simulink model "mainV02_36"  (R2016b)
settings: Solver=FixedStepAuto  StartTime=0.0  StopTime=inf  FixedStep=Ts  MaxStep=0.2  RelTol=1e-2
undefined symbols (not defined in the file): checks, deltae_degrees, deltafl_degrees, deltafr_degrees, deltar_degrees, deltat_1, deltat_2, deltat_3, deltat_4, deltat_5, Earth, F, ft, groundReaction, initialValues, LD, Light, m, MIL, Newton, Raphson, s, sigbuilder_block, Ts, WGS84
libraries: aerolibutil x19, simulink x16, aerolibtransform2 x7, aerolibasang x4, aerolib6dofsys x4, aerolib6dof2 x4, aerolibwind2 x3, aerolibbdyn x3, aerolibconvert2 x3, aerolibconvert x2, vrlib x2, aerolibatmos2 x1
(part 4 of 5)

== system mainV02_36/LIBIS Plant/Propulsion/8S 25C Battery ==
  note: ZIPPY Compact 5800mAh 8S 25C Lipo Pack
      |
      | Spec.
      | Capacity: 5800mAh
      | Voltage: 8S1P / 8 Cell / 29.6V
      | Discharge: 25C Constant / 35C Burst
      | Weight: 1025g (including wire, plug & case)
      | Dimensions: 167x46x64mm
      | Balance Plug: JST-XH
      | Discharge Plug: 5.5mm Bullet
  note: ZIPPY Compact 5800mAh 8S 25C Lipo Pack
      |
      | SKU
      | ZC.5800.8S.25
      | Weight(g):
      | 1020.00
      | Length:
      | 161.00
      | Width
      | 46.00
      | Height
      | 73.00
      | Capacity (mAh):
      | 5800.00
      | Discharge(c):
      | 25.00
      | Length-A(mm)
      | 167.00
      | Height-B(mm)
      | 46.00
      | Width-C(mm):
      | 64.00
      | Unit Weight (g):
      | 1020
      | Max Charge Rate(C)
      | 5.00
      | Watt Hour
      | 171.00
  note: Batería escogida: 8S 29.6V
  Battery_Capacity : Constant  Value=5.8
  Battery_Voltage : Constant  Value=29.6
  Max_discharge_rate : Constant  Value=145
  profundidad_descarga : Constant  Value=0.95
  rendimiento_bateria : Constant  Value=0.98
  C_battery : Outport  Unit=A*h
  deep_discharge_battery : Outport  Port=2  Unit=1
  V_battery : Outport  Port=3  Unit=V
  eta_battery : Outport  Port=4  Unit=1
  max_discharge_rate : Outport  Port=5  Unit=A*h
  wires:
  Battery_Voltage/1 -> V_battery/1
  Battery_Capacity/1 -> C_battery/1
  profundidad_descarga/1 -> deep_discharge_battery/1
  rendimiento_bateria/1 -> eta_battery/1
  Max_discharge_rate/1 -> max_discharge_rate/1

== system mainV02_36/LIBIS Plant/Propulsion/Variant_Motor_1 ==
  note: 1) Add Subsystem or Model blocks as valid variant choices.
      | 2) You cannot connect blocks at this level. At simulation, connectivity is automatically
      | determined, based on the active variant and port name matching.
  Vbattery : Inport
  Throttle : Inport  Port=2
  envData : Inport  Port=3
  plantData : Inport  Port=4
  mappedMotor_1 : Subsystem  VariantControl=mappedMotors==1
  noMappedMotor_1 : Subsystem  VariantControl=mappedMotors~=1
  Im : Outport
  Thrust : Outport  Port=2
  Thrust_moment : Outport  Port=3

== system mainV02_36/LIBIS Plant/Propulsion/Variant_Motor_2 ==
  note: 1) Add Subsystem or Model blocks as valid variant choices.
      | 2) You cannot connect blocks at this level. At simulation, connectivity is automatically
      | determined, based on the active variant and port name matching.
  Vbattery : Inport
  Throttle : Inport  Port=2
  envData : Inport  Port=3
  plantData : Inport  Port=4
  mappedMotor_2 : Subsystem  VariantControl=mappedMotors==1
  noMappedMotor_2 : Subsystem  VariantControl=mappedMotors~=1
  Im : Outport
  Thrust : Outport  Port=2
  Thrust_moment : Outport  Port=3

== system mainV02_36/LIBIS Plant/Propulsion/Variant_Motor_3 ==
  note: 1) Add Subsystem or Model blocks as valid variant choices.
      | 2) You cannot connect blocks at this level. At simulation, connectivity is automatically
      | determined, based on the active variant and port name matching.
  Vbattery : Inport
  Throttle : Inport  Port=2
  envData : Inport  Port=3
  plantData : Inport  Port=4
  mappedMotor_3 : Subsystem  VariantControl=mappedMotors==1
  noMappedMotor_3 : Subsystem  VariantControl=mappedMotors~=1
  Im : Outport
  Thrust : Outport  Port=2
  Thrust_moment : Outport  Port=3

== system mainV02_36/LIBIS Plant/Propulsion/Variant_Motor_4 ==
  note: 1) Add Subsystem or Model blocks as valid variant choices.
      | 2) You cannot connect blocks at this level. At simulation, connectivity is automatically
      | determined, based on the active variant and port name matching.
  Vbattery : Inport
  Throttle : Inport  Port=2
  envData : Inport  Port=3
  plantData : Inport  Port=4
  mappedMotor_4 : Subsystem  VariantControl=mappedMotors==1
  noMappedMotor_4 : Subsystem  VariantControl=mappedMotors~=1
  Im : Outport
  Thrust : Outport  Port=2
  Thrust_moment : Outport  Port=3

== system mainV02_36/LIBIS Plant/Propulsion/Variant_Motor_5 ==
  note: 1) Add Subsystem or Model blocks as valid variant choices.
      | 2) You cannot connect blocks at this level. At simulation, connectivity is automatically
      | determined, based on the active variant and port name matching.
  Vbattery : Inport
  Throttle : Inport  Port=2
  envData : Inport  Port=3
  plantData : Inport  Port=4
  mappedMotor_5 : Subsystem  VariantControl=mappedMotors==1
  noMappedMotor_5 : Subsystem  VariantControl=mappedMotors~=1
  Im : Outport
  Thrust : Outport  Port=2
  Thrust_moment : Outport  Port=3

== system mainV02_36/LIBIS Plant/Subsystem/calc alpha_dot ==
  q : Inport
  alpha,beta : Inport  Port=2
  Ab : Inport  Port=3
  Vw : Inport  Port=4
  Direction Cosine Matrix Body to Wind : aerolibtransform2/Direction Cosine Matrix Body to Wind
  Product1 : Product  Multiplication=Matrix(*)  SaturateOnIntegerOverflow=on  InputSameDT=on  OutDataTypeStr=Inherit: Same as first input
  Product2 : Product  Inputs=*/  SaturateOnIntegerOverflow=on  InputSameDT=on  OutDataTypeStr=Inherit: Same as first input
  Selector2 : Selector  IndexMode=Zero-based  InputPortWidth=3  IndexOptions=Index vector (dialog)  Indices=2  OutputSizes=1
  Selector3 : Selector  IndexMode=Zero-based  InputPortWidth=3  IndexOptions=Index vector (dialog)  Indices=0  OutputSizes=1
  Sum : Sum  Inputs=++|
  Transpose1 : Math  Operator=transpose  SaturateOnIntegerOverflow=on
  alpha_dot : Outport
  wires:
  Direction Cosine Matrix Body to Wind/1 -> Transpose1/1
  Transpose1/1 -> Product1/1
  Product1/1 -> Selector2/1
  Selector2/1 -> Product2/1
  Selector3/1 -> Product2/2
  Product2/1 -> Sum/2
  alpha,beta/1 -> Direction Cosine Matrix Body to Wind/1
  q/1 -> Sum/1
  Sum/1 -> alpha_dot/1
  Ab/1 -> Product1/2
  Vw/1 -> Selector3/1

== system mainV02_36/LIBIS Plant/alpha_dot, beta_dot/Subsystem ==
  beta : Inport  Unit=rad
  alpha : Inport  Port=2  Unit=rad
  V_body : Inport  Port=3  Unit=meter/s
  Omega_body : Inport  Port=4  Unit=rad/s
  Accel_body : Inport  Port=5  Unit=m/s^2
  Constant11 : Constant  Value=0
  Direction Cosine Matrix Body to Wind : aerolibtransform2/Direction Cosine Matrix Body to Wind
  Mux4 : Mux  Inputs=2
  Product1 : Product  Multiplication=Matrix(*)  SaturateOnIntegerOverflow=on  InputSameDT=on  OutDataTypeStr=Inherit: Same as first input
  Selector : Selector  InputPortWidth=3  IndexOptions=Index vector (dialog)  Indices=[2]  OutputSizes=1
  calc alpha_dot : Subsystem
  alpha_dot : Outport  Unit=rad/s
  beta_dot : Outport  Port=2
  wires:
  Direction Cosine Matrix Body to Wind/1 -> Product1/1
  Product1/1 -> calc alpha_dot/4(Vw)
  Mux4/1 -> Direction Cosine Matrix Body to Wind/1, calc alpha_dot/2(alpha,beta)
  Constant11/1 -> beta_dot/1  "beta_dot"
  alpha/1 -> Mux4/1
  Omega_body/1 -> Selector/1
  V_body/1 -> Product1/2
  Accel_body/1 -> calc alpha_dot/3(Ab)
  beta/1 -> Mux4/2
  calc alpha_dot/1(alpha_dot) -> alpha_dot/1
  Selector/1 -> calc alpha_dot/1(q)  "q"

== system mainV02_36/Sensors (Feedthrough)/IMU/Calculate DCM & Euler Angles ==
  "p q r " : Inport
  Rotation Angles to Direction Cosine Matrix : aerolibtransform2/Rotation Angles to Direction Cosine Matrix  rotationOrder=ZYX
  Selector : Selector  InputPortWidth=3  IndexOptions=Index vector (dialog)  Indices=[3 2 1]  OutputSizes=1
  phi theta psi : Integrator  InitialCondition=[initialValues.roll0 initialValues.pitch0 initialValues.yaw0]
  phidot thetadot psidot : aerolib6dofsys/DCM & Euler Angles (Euler)/phidot thetadot psidot
  DCMMeas : Outport
  EulerMeas : Outport  Port=2
  wires:
  Selector/1 -> Rotation Angles to Direction Cosine Matrix/1
  phi theta psi/1 -> EulerMeas/1, Selector/1, phidot thetadot psidot/2
  phidot thetadot psidot/1 -> phi theta psi/1
  "p q r "/1 -> phidot thetadot psidot/1
  Rotation Angles to Direction Cosine Matrix/1 -> DCMMeas/1

== system mainV02_36/Visualization/Euler to VR/Axis Angle Vector ==
  e0 : Inport
  2 : Gain  Gain=2  SaturateOnIntegerOverflow=on  OutDataTypeStr=Inherit: Same as input  ParamDataTypeStr=Inherit: Same as input
  Concatenate : Concatenate
  Constant : Constant  Value=[0 0 0]
  Demux : Demux  Outputs=[1 3 ]
  Product : Product  Inputs=*/  SaturateOnIntegerOverflow=on  InputSameDT=on  OutDataTypeStr=Inherit: Same as first input
  Switch : Switch  Criteria=u2 > Threshold
  Trigonometric Function : Trigonometry
  Trigonometric Function2 : Trigonometry  Operator=acos
  e0_norm : Outport
  wires:
  Demux/1 -> Trigonometric Function2/1
  Demux/2 -> Product/1
  Concatenate/1 -> e0_norm/1
  2/1 -> Concatenate/2
  Trigonometric Function/1 -> Switch/2, Product/2
  Trigonometric Function2/1 -> Trigonometric Function/1, 2/1
  e0/1 -> Demux/1
  Switch/1 -> Concatenate/1
  Product/1 -> Switch/1
  Constant/1 -> Switch/3

== system mainV02_36/Visualization/Euler to VR/Quaternion Normalization ==
  e0 : Inport
  1/2 : Gain  Gain=1/2  SaturateOnIntegerOverflow=on  OutDataTypeStr=Inherit: Same as input  ParamDataTypeStr=Inherit: Same as input
  Concatenate : Concatenate
  Demux : Demux  Outputs=[1 3]
  Product : Product  SaturateOnIntegerOverflow=on  InputSameDT=on  OutDataTypeStr=Inherit: Same as first input
  Trigonometric Function : Trigonometry
  Trigonometric Function1 : Trigonometry  Operator=cos
  e0_norm : Outport
  wires:
  Trigonometric Function1/1 -> Concatenate/1
  Demux/2 -> Product/2
  Demux/1 -> 1/2/1
  Concatenate/1 -> e0_norm/1
  Product/1 -> Concatenate/2
  Trigonometric Function/1 -> Product/1
  1/2/1 -> Trigonometric Function1/1, Trigonometric Function/1
  e0/1 -> Demux/1

== system mainV02_36/Visualization/Euler to VR/Quaternion Normalization1 ==
  e0 : Inport
  1/2 : Gain  Gain=1/2  SaturateOnIntegerOverflow=on  OutDataTypeStr=Inherit: Same as input  ParamDataTypeStr=Inherit: Same as input
  Concatenate : Concatenate
  Demux : Demux  Outputs=[1 3]
  Product : Product  SaturateOnIntegerOverflow=on  InputSameDT=on  OutDataTypeStr=Inherit: Same as first input
  Trigonometric Function : Trigonometry
  Trigonometric Function1 : Trigonometry  Operator=cos
  e0_norm : Outport
  wires:
  e0/1 -> Demux/1
  1/2/1 -> Trigonometric Function/1, Trigonometric Function1/1
  Trigonometric Function/1 -> Product/1
  Product/1 -> Concatenate/2
  Concatenate/1 -> e0_norm/1
  Demux/1 -> 1/2/1
  Demux/2 -> Product/2
  Trigonometric Function1/1 -> Concatenate/1

== system mainV02_36/Visualization/Euler to VR/Quaternion Normalization2 ==
  e0 : Inport
  1/2 : Gain  Gain=1/2  SaturateOnIntegerOverflow=on  OutDataTypeStr=Inherit: Same as input  ParamDataTypeStr=Inherit: Same as input
  Concatenate : Concatenate
  Demux : Demux  Outputs=[1 3]
  Product : Product  SaturateOnIntegerOverflow=on  InputSameDT=on  OutDataTypeStr=Inherit: Same as first input
  Trigonometric Function : Trigonometry
  Trigonometric Function1 : Trigonometry  Operator=cos
  e0_norm : Outport
  wires:
  Trigonometric Function1/1 -> Concatenate/1
  Demux/2 -> Product/2
  Demux/1 -> 1/2/1
  Concatenate/1 -> e0_norm/1
  Product/1 -> Concatenate/2
  Trigonometric Function/1 -> Product/1
  1/2/1 -> Trigonometric Function1/1, Trigonometric Function/1
  e0/1 -> Demux/1

== system mainV02_36/Visualization/Subsystem/Flightpath Angle ==
  Ve : Inport
  Constant : Constant  Value=eps
  Sum2 : Sum  Inputs=+  SaturateOnIntegerOverflow=on  InputSameDT=on  OutDataTypeStr=Inherit: Same as first input
  Switch : Switch  Criteria=u2 > Threshold
  product : Product  SaturateOnIntegerOverflow=on  InputSameDT=on  OutDataTypeStr=Inherit: Same as first input
  product1 : Product  Inputs=/*  SaturateOnIntegerOverflow=on  InputSameDT=on  OutDataTypeStr=Inherit: Same as first input
  rad-->deg4 : Gain  Gain=-1  SaturateOnIntegerOverflow=on  OutDataTypeStr=Inherit: Same as input  ParamDataTypeStr=Inherit: Same as input
  tangent : Trigonometry  Operator=atan
  u,v : Selector  IndexMode=Zero-based  InputPortWidth=3  IndexOptions=Index vector (dialog)  Indices=[0 1]  OutputSizes=1
  v : Sqrt  SaturateOnIntegerOverflow=on
  w : Selector  IndexMode=Zero-based  InputPortWidth=3  IndexOptions=Index vector (dialog)  Indices=2  OutputSizes=1
  gamma : Outport
  wires:
  Ve/1 -> w/1, u,v/1
  product/1 -> Sum2/1
  Sum2/1 -> v/1
  product1/1 -> tangent/1
  u,v/1 -> product/2, product/1
  w/1 -> rad-->deg4/1
  v/1 -> Switch/2, product1/1
  rad-->deg4/1 -> product1/2
  tangent/1 -> Switch/1
  Constant/1 -> Switch/3
  Switch/1 -> gamma/1

== system mainV02_36/LIBIS Plant/Propulsion/Variant_Motor_1/mappedMotor_1 ==
  Vbattery : Inport
  Throttle : Inport  Port=2
  envData : Inport  Port=3
  plantData : Inport  Port=4
  3x3 Cross Product : aerolibutil/3x3 Cross Product
  Bus Selector : BusSelector  OutputSignals=V_body,CG,LLA.Altitude_m
  Bus Selector1 : BusSelector  OutputSignals=windVelocity
  Constant{1..4} (4 alike) : Constant  Value=0
  ESC_1 : Subsystem
  Motor and Propeller Coupling_1 : Subsystem
  Mux : Mux  Inputs=3
  Mux1 : Mux  Inputs=3
  Selector1 : Selector  InputPortWidth=3  IndexOptions=Index vector (dialog)  Indices=[1]  OutputSizes=1
  Selector2 : Selector  InputPortWidth=3  IndexOptions=Index vector (dialog)  Indices=[1]  OutputSizes=1
  Sum : Sum  Inputs=|+-
  Sum1 : Sum  Inputs=+-|
  Sum2 : Sum  Inputs=|++
  Terminator : Terminator
  Torque : Subsystem
  "motor2 position " : Constant  Value=LD.Propulsion.motor1.Position
  Im : Outport
  Thrust : Outport  Port=2
  Thrust_moment : Outport  Port=3
  wires:
  Vbattery/1 -> ESC_1/1(V_battery)
  ESC_1/1(V_ESC) -> Motor and Propeller Coupling_1/1(Voltage)  "V_ESC"
  Mux/1 -> Thrust/1, 3x3 Cross Product/2  "Thrust_vector"
  Throttle/1 -> ESC_1/2(Throttle)
  Constant1/1 -> Mux/2
  Sum1/1 -> 3x3 Cross Product/1  "arm"
  Motor and Propeller Coupling_1/3(Current) -> Im/1
  Bus Selector/2 -> [CG]  "<CG>"
  Bus Selector/3 -> [Altitude]  "<Altitude_m>"
  Bus Selector1/1 -> [V_wind]  "<windVelocity>"
  [CG] -> Sum1/2
  Selector2/1 -> Sum/1
  Selector1/1 -> Sum/2
  plantData/1 -> Bus Selector/1
  [V_body] -> Selector2/1
  Motor and Propeller Coupling_1/1(Thrust) -> Mux/1  "Thrust_scalar"
  [Altitude] -> Motor and Propeller Coupling_1/2(Height)
  "motor2 position "/1 -> Sum1/1
  [V_wind] -> Selector1/1
  Constant2/1 -> Mux/3
  Bus Selector/1 -> [V_body]  "<V_body>"
  envData/1 -> Bus Selector1/1
  Motor and Propeller Coupling_1/2(Power) -> Terminator/1
  Sum/1 -> Torque/2(Vflight), Motor and Propeller Coupling_1/3(Vflight)
  Mux1/1 -> Sum2/2  "Torque_vector"
  Constant3/1 -> Mux1/2
  Sum2/1 -> Thrust_moment/1
  3x3 Cross Product/1 -> Sum2/1
  Motor and Propeller Coupling_1/4(RPM) -> Torque/1(RPM)  "RPM"
  Constant4/1 -> Mux1/3
  Torque/1(Torque) -> Mux1/1

== system mainV02_36/LIBIS Plant/Propulsion/Variant_Motor_1/noMappedMotor_1 ==
  Vbattery : Inport
  Throttle : Inport  Port=2
  envData : Inport  Port=3
  plantData : Inport  Port=4
  3x3 Cross Product : aerolibutil/3x3 Cross Product
  Algebraic Constraint : simulink/Math Operations/Algebraic Constraint  z0=0
  Bus Selector : BusSelector  OutputSignals=V_body,CG
  Bus Selector1 : BusSelector  OutputSignals=windVelocity,AirDensity
  Constant{1..4} (4 alike) : Constant  Value=0
  ESC_1 : Subsystem
  Motor_1 : Subsystem
  Mux : Mux  Inputs=3
  Mux1 : Mux  Inputs=3
  Propeller_1 : Subsystem
  Selector1 : Selector  InputPortWidth=3  IndexOptions=Index vector (dialog)  Indices=[1]  OutputSizes=1
  Selector3 : Selector  InputPortWidth=3  IndexOptions=Index vector (dialog)  Indices=[1]  OutputSizes=1
  Sum : Sum  Inputs=|+-
  Sum1 : Sum  Inputs=+|-
  Sum2 : Sum  Inputs=|+-
  Sum3 : Sum  Inputs=++|
  Torque : Subsystem
  "motor1 position " : Constant  Value=LD.Propulsion.motor1.Position
  Im : Outport
  Thrust : Outport  Port=2
  Thrust_moment : Outport  Port=3
  wires:
  Throttle/1 -> ESC_1/2(Throttle)
  Vbattery/1 -> ESC_1/1(V_battery)
  Motor_1/2(Peje) -> Sum/1  "P_available"
  Motor_1/1(RPM) -> Torque/1(RPM), Propeller_1/1(RPM)  "RPM"
  "motor1 position "/1 -> Sum1/1
  Sum/1 -> Algebraic Constraint/1  "P_error"
  Algebraic Constraint/1 -> Im/1, Motor_1/2(Im)  "Im"
  Sum1/1 -> 3x3 Cross Product/1  "arm"
  Propeller_1/1(P_needed) -> Sum/2  "P_needed"
  Mux/1 -> Thrust/1, 3x3 Cross Product/2  "Thrust_vector1"
  Propeller_1/2(Thrust) -> Mux/1  "Thrust_scalar"
  Constant1/1 -> Mux/2
  Constant2/1 -> Mux/3
  [CG] -> Sum1/2
  ESC_1/1(V_ESC) -> Motor_1/1(V_ESC)
  plantData/1 -> Bus Selector/1
  Bus Selector/1 -> [V_body]  "<V_body>"
  Bus Selector/2 -> [CG]  "<CG>"
  [V_body] -> Selector3/1
  [V_wind] -> Selector1/1
  Selector1/1 -> Sum2/2
  Selector3/1 -> Sum2/1
  envData/1 -> Bus Selector1/1
  Bus Selector1/1 -> [V_wind]  "<windVelocity>"
  Bus Selector1/2 -> [AirDensity]  "<AirDensity>"
  [AirDensity] -> Propeller_1/3(airDensity)
  Constant3/1 -> Mux1/2
  Constant4/1 -> Mux1/3
  Torque/1(Torque) -> Mux1/1
  Mux1/1 -> Sum3/1  "Torque_vector"
  Sum3/1 -> Thrust_moment/1
  3x3 Cross Product/1 -> Sum3/2
  Sum2/1 -> Propeller_1/2(V_flight), Torque/2(Vflight)

== system mainV02_36/LIBIS Plant/Propulsion/Variant_Motor_2/mappedMotor_2 ==
  Vbattery : Inport
  Throttle : Inport  Port=2
  envData : Inport  Port=3
  plantData : Inport  Port=4
  3x3 Cross Product : aerolibutil/3x3 Cross Product
  Bus Selector : BusSelector  OutputSignals=V_body,CG,LLA.Altitude_m
  Bus Selector1 : BusSelector  OutputSignals=windVelocity
  Constant{1..4} (4 alike) : Constant  Value=0
  ESC_2 : Subsystem
  Motor and Propeller Coupling_2 : Subsystem
  Mux : Mux  Inputs=3
  Mux1 : Mux  Inputs=3
  Selector1 : Selector  InputPortWidth=3  IndexOptions=Index vector (dialog)  Indices=[3]  OutputSizes=1
  Selector2 : Selector  InputPortWidth=3  IndexOptions=Index vector (dialog)  Indices=[3]  OutputSizes=1
  Sum : Sum  Inputs=|+-
  Sum1 : Sum  Inputs=+-|
  Sum2 : Sum  Inputs=|++
  Terminator : Terminator
  Torque : Subsystem
  Unary Minus : UnaryMinus
  "motor2 position " : Constant  Value=LD.Propulsion.motor2.Position
  Im : Outport
  Thrust : Outport  Port=2
  Thrust_moment : Outport  Port=3
  wires:
  ESC_2/1(V_ESC) -> Motor and Propeller Coupling_2/1(Voltage)  "V_ESC"
  [V_body] -> Selector2/1
  Vbattery/1 -> ESC_2/1(V_battery)
  Bus Selector/1 -> [V_body]  "<V_body>"
  Motor and Propeller Coupling_2/1(Thrust) -> Unary Minus/1  "Thrust_scalar"
  Unary Minus/1 -> Mux/3
  Bus Selector/3 -> [Altitude]  "<Altitude_m>"
  [CG] -> Sum1/2
  "motor2 position "/1 -> Sum1/1
  Motor and Propeller Coupling_2/3(Current) -> Im/1
  Sum1/1 -> 3x3 Cross Product/1  "arm"
  Constant2/1 -> Mux/1
  Mux/1 -> Thrust/1, 3x3 Cross Product/2  "Thrust_vector"
  Constant1/1 -> Mux/2
  Throttle/1 -> ESC_2/2(Throttle)
  plantData/1 -> Bus Selector/1
  Bus Selector/2 -> [CG]  "<CG>"
  [V_wind] -> Selector1/1
  [Altitude] -> Motor and Propeller Coupling_2/2(Height)
  Sum/1 -> Torque/2(Vflight), Motor and Propeller Coupling_2/3(Vflight)
  Motor and Propeller Coupling_2/4(RPM) -> Torque/1(RPM)
  Motor and Propeller Coupling_2/2(Power) -> Terminator/1
  envData/1 -> Bus Selector1/1
  Selector1/1 -> Sum/2
  Bus Selector1/1 -> [V_wind]  "<windVelocity>"
  Selector2/1 -> Sum/1
  Constant4/1 -> Mux1/1
  Mux1/1 -> Sum2/2  "Torque_vector"
  Constant3/1 -> Mux1/2
  Sum2/1 -> Thrust_moment/1
  3x3 Cross Product/1 -> Sum2/1
  Torque/1(Torque) -> Mux1/3  "Torque"

== system mainV02_36/LIBIS Plant/Propulsion/Variant_Motor_2/noMappedMotor_2 ==
  Vbattery : Inport
  Throttle : Inport  Port=2
  envData : Inport  Port=3
  plantData : Inport  Port=4
  3x3 Cross Product : aerolibutil/3x3 Cross Product
  Algebraic Constraint : simulink/Math Operations/Algebraic Constraint  z0=0
  Bus Selector : BusSelector  OutputSignals=V_body,CG
  Bus Selector1 : BusSelector  OutputSignals=windVelocity,AirDensity
  Constant{1..4} (4 alike) : Constant  Value=0
  ESC_2 : Subsystem
  Motor_2 : Subsystem
  Mux : Mux  Inputs=3
  Mux1 : Mux  Inputs=3
  Propeller_2 : Subsystem
  Selector1 : Selector  InputPortWidth=3  IndexOptions=Index vector (dialog)  Indices=[3]  OutputSizes=1
  Selector3 : Selector  InputPortWidth=3  IndexOptions=Index vector (dialog)  Indices=[3]  OutputSizes=1
  Sum : Sum  Inputs=|+-
  Sum1 : Sum  Inputs=+|-
  Sum2 : Sum  Inputs=|+-
  Sum3 : Sum  Inputs=++|
  Torque : Subsystem
  Unary Minus : UnaryMinus
  "motor2 position " : Constant  Value=LD.Propulsion.motor2.Position
  Im : Outport
  Thrust : Outport  Port=2
  Thrust_moment : Outport  Port=3
  wires:
  [AirDensity] -> Propeller_2/3(airDensity)
  Sum1/1 -> 3x3 Cross Product/1  "arm"
  Throttle/1 -> ESC_2/2(Throttle)
  Mux/1 -> Thrust/1, 3x3 Cross Product/2  "Thrust_vector1"
  Sum/1 -> Algebraic Constraint/1  "P_error"
  Propeller_2/1(P_needed) -> Sum/2  "P_needed"
  Vbattery/1 -> ESC_2/1(V_battery)
  Motor_2/1(RPM) -> Torque/1(RPM), Propeller_2/1(RPM)  "RPM"
  [CG] -> Sum1/2
  Constant2/1 -> Mux/1
  plantData/1 -> Bus Selector/1
  Motor_2/2(Peje) -> Sum/1  "P_available"
  Bus Selector/1 -> [V_body]  "<V_body>"
  Constant1/1 -> Mux/2
  Bus Selector/2 -> [CG]  "<CG>"
  "motor2 position "/1 -> Sum1/1
  ESC_2/1(V_ESC) -> Motor_2/1(V_ESC)  "V_ESC"
  Algebraic Constraint/1 -> Im/1, Motor_2/2(Im)  "Im"
  Propeller_2/2(Thrust) -> Unary Minus/1  "Thrust_scalar"
  Unary Minus/1 -> Mux/3
  [V_body] -> Selector3/1
  [V_wind] -> Selector1/1
  Sum2/1 -> Torque/2(Vflight), Propeller_2/2(V_flight)
  Selector1/1 -> Sum2/2
  Selector3/1 -> Sum2/1
  envData/1 -> Bus Selector1/1
  Bus Selector1/1 -> [V_wind]  "<windVelocity>"
  Bus Selector1/2 -> [AirDensity]  "<AirDensity>"
  Constant4/1 -> Mux1/1
  Constant3/1 -> Mux1/2
  Torque/1(Torque) -> Mux1/3  "Torque"
  3x3 Cross Product/1 -> Sum3/2
  Sum3/1 -> Thrust_moment/1
  Mux1/1 -> Sum3/1  "Torque_vector"

== system mainV02_36/LIBIS Plant/Propulsion/Variant_Motor_3/mappedMotor_3 ==
  Vbattery : Inport
  Throttle : Inport  Port=2
  envData : Inport  Port=3
  plantData : Inport  Port=4
  3x3 Cross Product : aerolibutil/3x3 Cross Product
  Bus Selector : BusSelector  OutputSignals=V_body,CG,LLA.Altitude_m
  Bus Selector1 : BusSelector  OutputSignals=windVelocity
  Constant{1..4} (4 alike) : Constant  Value=0
  ESC_3 : Subsystem
  Motor and Propeller Coupling_3 : Subsystem
  Mux : Mux  Inputs=3
  Mux1 : Mux  Inputs=3
  Selector1 : Selector  InputPortWidth=3  IndexOptions=Index vector (dialog)  Indices=[3]  OutputSizes=1
  Selector2 : Selector  InputPortWidth=3  IndexOptions=Index vector (dialog)  Indices=[3]  OutputSizes=1
  Sum : Sum  Inputs=|+-
  Sum1 : Sum  Inputs=+-|
  Sum2 : Sum  Inputs=|++
  Terminator : Terminator
  Torque : Subsystem
  Unary Minus : UnaryMinus
  Unary Minus1 : UnaryMinus
  "motor2 position " : Constant  Value=LD.Propulsion.motor3.Position
  Im : Outport
  Thrust : Outport  Port=2
  Thrust_moment : Outport  Port=3
  wires:
  ESC_3/1(V_ESC) -> Motor and Propeller Coupling_3/1(Voltage)  "V_ESC"
  [V_wind] -> Selector1/1
  Motor and Propeller Coupling_3/1(Thrust) -> Unary Minus/1  "Thrust_scalar"
  Motor and Propeller Coupling_3/2(Power) -> Terminator/1
  Throttle/1 -> ESC_3/2(Throttle)
  Selector2/1 -> Sum/1
  Selector1/1 -> Sum/2
  Mux/1 -> Thrust/1, 3x3 Cross Product/2  "Thrust_vector"
  Motor and Propeller Coupling_3/3(Current) -> Im/1
  [V_body] -> Selector2/1
  plantData/1 -> Bus Selector/1
  Constant1/1 -> Mux/2
  envData/1 -> Bus Selector1/1
  Sum1/1 -> 3x3 Cross Product/1  "arm"
  Bus Selector/1 -> [V_body]  "<V_body>"
  Bus Selector/2 -> [CG]  "<CG>"
  Constant2/1 -> Mux/1
  Unary Minus/1 -> Mux/3
  [Altitude] -> Motor and Propeller Coupling_3/2(Height)
  "motor2 position "/1 -> Sum1/1
  Bus Selector1/1 -> [V_wind]  "<windVelocity>"
  [CG] -> Sum1/2
  Vbattery/1 -> ESC_3/1(V_battery)
  Bus Selector/3 -> [Altitude]  "<Altitude_m>"
  Sum/1 -> Torque/2(Vflight), Motor and Propeller Coupling_3/3(Vflight)
  Motor and Propeller Coupling_3/4(RPM) -> Torque/1(RPM)  "RPM"
  Constant4/1 -> Mux1/1
  Mux1/1 -> Sum2/2  "Torque_vector"
  Constant3/1 -> Mux1/2
  Sum2/1 -> Thrust_moment/1
  3x3 Cross Product/1 -> Sum2/1
  Torque/1(Torque) -> Unary Minus1/1
  Unary Minus1/1 -> Mux1/3

== system mainV02_36/LIBIS Plant/Propulsion/Variant_Motor_3/noMappedMotor_3 ==
  Vbattery : Inport
  Throttle : Inport  Port=2
  envData : Inport  Port=3
  plantData : Inport  Port=4
  3x3 Cross Product : aerolibutil/3x3 Cross Product
  Algebraic Constraint : simulink/Math Operations/Algebraic Constraint  z0=0
  Bus Selector : BusSelector  OutputSignals=V_body,CG
  Bus Selector1 : BusSelector  OutputSignals=windVelocity,AirDensity
  Constant{1..4} (4 alike) : Constant  Value=0
  ESC_3 : Subsystem
  Motor_3 : Subsystem
  Mux : Mux  Inputs=3
  Mux1 : Mux  Inputs=3
  Propeller_3 : Subsystem
  Selector1 : Selector  InputPortWidth=3  IndexOptions=Index vector (dialog)  Indices=[3]  OutputSizes=1
  Selector3 : Selector  InputPortWidth=3  IndexOptions=Index vector (dialog)  Indices=[3]  OutputSizes=1
  Sum : Sum  Inputs=|+-
  Sum1 : Sum  Inputs=+|-
  Sum2 : Sum  Inputs=|+-
  Sum3 : Sum  Inputs=++|
  Torque : Subsystem
  Unary Minus : UnaryMinus
  Unary Minus1 : UnaryMinus
  "motor3 position " : Constant  Value=LD.Propulsion.motor3.Position
  Im : Outport
  Thrust : Outport  Port=2
  Thrust_moment : Outport  Port=3
  wires:
  Throttle/1 -> ESC_3/2(Throttle)
  Vbattery/1 -> ESC_3/1(V_battery)
  Propeller_3/2(Thrust) -> Unary Minus/1  "Thrust_scalar"
  Motor_3/2(Peje) -> Sum/1  "P_available"
  Sum1/1 -> 3x3 Cross Product/1  "arm"
  "motor3 position "/1 -> Sum1/1
  Mux/1 -> Thrust/1, 3x3 Cross Product/2  "Thrust_vector1"
  Constant1/1 -> Mux/2
  Constant2/1 -> Mux/1
  Algebraic Constraint/1 -> Im/1, Motor_3/2(Im)  "Im"
  [CG] -> Sum1/2
  ESC_3/1(V_ESC) -> Motor_3/1(V_ESC)
  Sum/1 -> Algebraic Constraint/1  "P_error"
  Unary Minus/1 -> Mux/3
  Propeller_3/1(P_needed) -> Sum/2  "P_needed"
  plantData/1 -> Bus Selector/1
  Bus Selector/1 -> [V_body]  "<V_body>"
  Bus Selector/2 -> [CG]  "<CG>"
  envData/1 -> Bus Selector1/1
  Bus Selector1/1 -> [V_wind]  "<windVelocity>"
  Bus Selector1/2 -> [AirDensity]  "<AirDensity>"
  [V_body] -> Selector3/1
  [V_wind] -> Selector1/1
  Selector1/1 -> Sum2/2
  Selector3/1 -> Sum2/1
  [AirDensity] -> Propeller_3/3(airDensity)
  Motor_3/1(RPM) -> Torque/1(RPM), Propeller_3/1(RPM)  "RPM"
  Sum2/1 -> Torque/2(Vflight), Propeller_3/2(V_flight)
  Constant4/1 -> Mux1/1
  Constant3/1 -> Mux1/2
  Torque/1(Torque) -> Mux1/3  "Torque"
  Sum3/1 -> Thrust_moment/1
  3x3 Cross Product/1 -> Sum3/2
  Unary Minus1/1 -> Sum3/1
  Mux1/1 -> Unary Minus1/1  "Torque_vector"

== system mainV02_36/LIBIS Plant/Propulsion/Variant_Motor_4/mappedMotor_4 ==
  Vbattery : Inport
  Throttle : Inport  Port=2
  envData : Inport  Port=3
  plantData : Inport  Port=4
  3x3 Cross Product : aerolibutil/3x3 Cross Product
  Bus Selector : BusSelector  OutputSignals=V_body,CG,LLA.Altitude_m
  Bus Selector1 : BusSelector  OutputSignals=windVelocity
  Constant{1..4} (4 alike) : Constant  Value=0
  ESC_4 : Subsystem
  Motor and Propeller Coupling_4 : Subsystem
  Mux : Mux  Inputs=3
  Mux1 : Mux  Inputs=3
  Selector1 : Selector  InputPortWidth=3  IndexOptions=Index vector (dialog)  Indices=[3]  OutputSizes=1
  Selector2 : Selector  InputPortWidth=3  IndexOptions=Index vector (dialog)  Indices=[3]  OutputSizes=1
  Sum : Sum  Inputs=|+-
  Sum1 : Sum  Inputs=+-|
  Sum2 : Sum  Inputs=|++
  Terminator : Terminator
  Torque : Subsystem
  Unary Minus : UnaryMinus
  "motor2 position " : Constant  Value=LD.Propulsion.motor4.Position
  Im : Outport
  Thrust : Outport  Port=2
  Thrust_moment : Outport  Port=3
  wires:
  Constant1/1 -> Mux/2
  ESC_4/1(V_ESC) -> Motor and Propeller Coupling_4/1(Voltage)  "V_ESC"
  plantData/1 -> Bus Selector/1
  Sum1/1 -> 3x3 Cross Product/1  "arm"
  Unary Minus/1 -> Mux/3
  Constant2/1 -> Mux/1
  Bus Selector/3 -> [Altitude]  "<Altitude_m>"
  [CG] -> Sum1/2
  Bus Selector/1 -> [V_body]  "<V_body>"
  Mux/1 -> Thrust/1, 3x3 Cross Product/2  "Thrust_vector"
  Throttle/1 -> ESC_4/2(Throttle)
  Vbattery/1 -> ESC_4/1(V_battery)
  Bus Selector/2 -> [CG]  "<CG>"
  Motor and Propeller Coupling_4/1(Thrust) -> Unary Minus/1  "Thrust_scalar"
  Bus Selector1/1 -> [V_wind]  "<windVelocity>"
  [V_wind] -> Selector1/1
  "motor2 position "/1 -> Sum1/1
  envData/1 -> Bus Selector1/1
  Selector1/1 -> Sum/2
  Motor and Propeller Coupling_4/2(Power) -> Terminator/1
  [V_body] -> Selector2/1
  Selector2/1 -> Sum/1
  Motor and Propeller Coupling_4/3(Current) -> Im/1
  [Altitude] -> Motor and Propeller Coupling_4/2(Height)
  Sum/1 -> Torque/2(Vflight), Motor and Propeller Coupling_4/3(Vflight)
  Motor and Propeller Coupling_4/4(RPM) -> Torque/1(RPM)  "RPM"
  Constant4/1 -> Mux1/1
  Mux1/1 -> Sum2/2  "Torque_vector"
  Constant3/1 -> Mux1/2
  Sum2/1 -> Thrust_moment/1
  3x3 Cross Product/1 -> Sum2/1
  Torque/1(Torque) -> Mux1/3  "Torque"

== system mainV02_36/LIBIS Plant/Propulsion/Variant_Motor_4/noMappedMotor_4 ==
  Vbattery : Inport
  Throttle : Inport  Port=2
  envData : Inport  Port=3
  plantData : Inport  Port=4
  3x3 Cross Product : aerolibutil/3x3 Cross Product
  Algebraic Constraint : simulink/Math Operations/Algebraic Constraint  z0=0
  Bus Selector : BusSelector  OutputSignals=V_body,CG
  Bus Selector1 : BusSelector  OutputSignals=windVelocity,AirDensity
  Constant{1..4} (4 alike) : Constant  Value=0
  ESC_4 : Subsystem
  Motor_4 : Subsystem
  Mux : Mux  Inputs=3
  Mux1 : Mux  Inputs=3
  Propeller_4 : Subsystem
  Selector1 : Selector  InputPortWidth=3  IndexOptions=Index vector (dialog)  Indices=[3]  OutputSizes=1
  Selector3 : Selector  InputPortWidth=3  IndexOptions=Index vector (dialog)  Indices=[3]  OutputSizes=1
  Sum : Sum  Inputs=|+-
  Sum1 : Sum  Inputs=+|-
  Sum2 : Sum  Inputs=|+-
  Sum3 : Sum  Inputs=++|
  Torque : Subsystem
  Unary Minus : UnaryMinus
  "motor4 position " : Constant  Value=LD.Propulsion.motor4.Position
  Im : Outport
  Thrust : Outport  Port=2
  Thrust_moment : Outport  Port=3
  wires:
  Constant1/1 -> Mux/2
  Throttle/1 -> ESC_4/2(Throttle)
  Motor_4/2(Peje) -> Sum/1  "P_available"
  Sum/1 -> Algebraic Constraint/1  "P_error"
  "motor4 position "/1 -> Sum1/1
  Algebraic Constraint/1 -> Im/1, Motor_4/2(Im)  "Im"
  Propeller_4/1(P_needed) -> Sum/2  "P_needed"
  Sum1/1 -> 3x3 Cross Product/1  "arm"
  Vbattery/1 -> ESC_4/1(V_battery)
  Mux/1 -> Thrust/1, 3x3 Cross Product/2  "Thrust_vector1"
  Constant2/1 -> Mux/1
  Propeller_4/2(Thrust) -> Unary Minus/1  "Thrust_scalar"
  Unary Minus/1 -> Mux/3
  [CG] -> Sum1/2
  ESC_4/1(V_ESC) -> Motor_4/1(V_ESC)
  plantData/1 -> Bus Selector/1
  Bus Selector/1 -> [V_body]  "<V_body>"
  Bus Selector/2 -> [CG]  "<CG>"
  [V_body] -> Selector3/1
  [V_wind] -> Selector1/1
  Selector1/1 -> Sum2/2
  Selector3/1 -> Sum2/1
  envData/1 -> Bus Selector1/1
  Bus Selector1/1 -> [V_wind]  "<windVelocity>"
  Bus Selector1/2 -> [AirDensity]  "<AirDensity>"
  [AirDensity] -> Propeller_4/3(airDensity)
  Motor_4/1(RPM) -> Torque/1(RPM), Propeller_4/1(RPM)  "RPM"
  Sum2/1 -> Torque/2(Vflight), Propeller_4/2(V_flight)
  Constant4/1 -> Mux1/1
  Constant3/1 -> Mux1/2
  Torque/1(Torque) -> Mux1/3  "Torque"
  Mux1/1 -> Sum3/1  "Torque_vector"
  3x3 Cross Product/1 -> Sum3/2
  Sum3/1 -> Thrust_moment/1

== system mainV02_36/LIBIS Plant/Propulsion/Variant_Motor_5/mappedMotor_5 ==
  Vbattery : Inport
  Throttle : Inport  Port=2
  envData : Inport  Port=3
  plantData : Inport  Port=4
  3x3 Cross Product : aerolibutil/3x3 Cross Product
  Bus Selector : BusSelector  OutputSignals=V_body,CG,LLA.Altitude_m
  Bus Selector1 : BusSelector  OutputSignals=windVelocity
  Constant{1..4} (4 alike) : Constant  Value=0
  ESC_5 : Subsystem
  Motor and Propeller Coupling_5 : Subsystem
  Mux : Mux  Inputs=3
  Mux1 : Mux  Inputs=3
  Selector1 : Selector  InputPortWidth=3  IndexOptions=Index vector (dialog)  Indices=[3]  OutputSizes=1
  Selector2 : Selector  InputPortWidth=3  IndexOptions=Index vector (dialog)  Indices=[3]  OutputSizes=1
  Sum : Sum  Inputs=|+-
  Sum1 : Sum  Inputs=+-|  InputSameDT=on
  Sum2 : Sum  Inputs=|++
  Terminator : Terminator
  Torque : Subsystem
  Unary Minus : UnaryMinus
  Unary Minus1 : UnaryMinus
  "motor2 position " : Constant  Value=LD.Propulsion.motor5.Position
  Im : Outport
  Thrust : Outport  Port=2
  Thrust_moment : Outport  Port=3
  wires:
  Throttle/1 -> ESC_5/2(Throttle)
  Vbattery/1 -> ESC_5/1(V_battery)
  Selector2/1 -> Sum/1
  Selector1/1 -> Sum/2
  [CG] -> Sum1/2
  Bus Selector/3 -> [Altitude]  "<Altitude_m>"
  envData/1 -> Bus Selector1/1
  [Altitude] -> Motor and Propeller Coupling_5/2(Height)
  Bus Selector/2 -> [CG]  "<CG>"
  Motor and Propeller Coupling_5/3(Current) -> Im/1
  plantData/1 -> Bus Selector/1
  Unary Minus/1 -> Mux/3
  "motor2 position "/1 -> Sum1/1
  [V_body] -> Selector2/1
  Bus Selector1/1 -> [V_wind]  "<windVelocity>"
  [V_wind] -> Selector1/1
  Motor and Propeller Coupling_5/2(Power) -> Terminator/1
  Constant1/1 -> Mux/2
  ESC_5/1(V_ESC) -> Motor and Propeller Coupling_5/1(Voltage)  "V_ESC"
  Mux/1 -> Thrust/1, 3x3 Cross Product/2  "Thrust_vector"
  Motor and Propeller Coupling_5/1(Thrust) -> Unary Minus/1  "Thrust_scalar"
  Constant2/1 -> Mux/1
  Sum1/1 -> 3x3 Cross Product/1  "arm"
  Bus Selector/1 -> [V_body]  "<V_body>"
  Sum/1 -> Torque/2(Vflight), Motor and Propeller Coupling_5/3(Vflight)
  Motor and Propeller Coupling_5/4(RPM) -> Torque/1(RPM)  "RPM"
  Constant4/1 -> Mux1/1
  Mux1/1 -> Sum2/2  "Torque_vector"
  Constant3/1 -> Mux1/2
  Sum2/1 -> Thrust_moment/1
  3x3 Cross Product/1 -> Sum2/1
  Torque/1(Torque) -> Unary Minus1/1
  Unary Minus1/1 -> Mux1/3

== system mainV02_36/LIBIS Plant/Propulsion/Variant_Motor_5/noMappedMotor_5 ==
  Vbattery : Inport
  Throttle : Inport  Port=2
  envData : Inport  Port=3
  plantData : Inport  Port=4
  3x3 Cross Product : aerolibutil/3x3 Cross Product
  Algebraic Constraint : simulink/Math Operations/Algebraic Constraint  z0=0.1
  Bus Selector : BusSelector  OutputSignals=V_body,CG
  Bus Selector1 : BusSelector  OutputSignals=windVelocity,AirDensity
  Constant{1..4} (4 alike) : Constant  Value=0
  ESC_5 : Subsystem
  Motor_5 : Subsystem
  Mux : Mux  Inputs=3
  Mux1 : Mux  Inputs=3
  Propeller_5 : Subsystem
  Selector1 : Selector  InputPortWidth=3  IndexOptions=Index vector (dialog)  Indices=[3]  OutputSizes=1
  Selector3 : Selector  InputPortWidth=3  IndexOptions=Index vector (dialog)  Indices=[3]  OutputSizes=1
  Sum : Sum  Inputs=|+-
  Sum1 : Sum  Inputs=+|-
  Sum2 : Sum  Inputs=|+-
  Sum3 : Sum  Inputs=++|
  Torque : Subsystem
  Unary Minus : UnaryMinus
  Unary Minus1 : UnaryMinus
  "motor5 position " : Constant  Value=LD.Propulsion.motor5.Position
  Im : Outport
  Thrust : Outport  Port=2
  Thrust_moment : Outport  Port=3
  wires:
  ESC_5/1(V_ESC) -> Motor_5/1(V_ESC)
  Unary Minus/1 -> Mux/3
  Propeller_5/2(Thrust) -> Unary Minus/1  "Thrust_scalar"
  Motor_5/2(Peje) -> Sum/1  "P_available"
  Throttle/1 -> ESC_5/2(Throttle)
  Propeller_5/1(P_needed) -> Sum/2  "P_needed"
  Algebraic Constraint/1 -> Im/1, Motor_5/2(Im)  "Im"
  Vbattery/1 -> ESC_5/1(V_battery)
  Sum/1 -> Algebraic Constraint/1  "P_error"
  "motor5 position "/1 -> Sum1/1
  Sum1/1 -> 3x3 Cross Product/1  "arm"
  Mux/1 -> Thrust/1, 3x3 Cross Product/2  "Thrust_vector1"
  [CG] -> Sum1/2
  Constant1/1 -> Mux/2
  Constant2/1 -> Mux/1
  plantData/1 -> Bus Selector/1
  Bus Selector/1 -> [V_body]  "<V_body>"
  Bus Selector/2 -> [CG]  "<CG>"
  [V_body] -> Selector3/1
  [V_wind] -> Selector1/1
  Selector1/1 -> Sum2/2
  Selector3/1 -> Sum2/1
  envData/1 -> Bus Selector1/1
  Bus Selector1/1 -> [V_wind]  "<windVelocity>"
  Bus Selector1/2 -> [AirDensity]  "<AirDensity>"
  [AirDensity] -> Propeller_5/3(airDensity)
  Motor_5/1(RPM) -> Torque/1(RPM), Propeller_5/1(RPM)  "RPM"
  Sum2/1 -> Torque/2(Vflight), Propeller_5/2(V_flight)
  Constant4/1 -> Mux1/1
  Constant3/1 -> Mux1/2
  Torque/1(Torque) -> Mux1/3  "Torque"
  Unary Minus1/1 -> Sum3/1
  Mux1/1 -> Unary Minus1/1  "Torque_vector"
  Sum3/1 -> Thrust_moment/1
  3x3 Cross Product/1 -> Sum3/2

== system mainV02_36/LIBIS Plant/alpha_dot, beta_dot/Subsystem/calc alpha_dot ==
  q : Inport
  alpha,beta : Inport  Port=2
  Ab : Inport  Port=3
  Vw : Inport  Port=4
  Direction Cosine Matrix Body to Wind : aerolibtransform2/Direction Cosine Matrix Body to Wind
  Product1 : Product  Multiplication=Matrix(*)  SaturateOnIntegerOverflow=on  InputSameDT=on  OutDataTypeStr=Inherit: Same as first input
  Product2 : Product  Inputs=*/  SaturateOnIntegerOverflow=on  InputSameDT=on  OutDataTypeStr=Inherit: Same as first input
  Selector2 : Selector  IndexMode=Zero-based  InputPortWidth=3  IndexOptions=Index vector (dialog)  Indices=2  OutputSizes=1
  Selector3 : Selector  IndexMode=Zero-based  InputPortWidth=3  IndexOptions=Index vector (dialog)  Indices=0  OutputSizes=1
  Sum : Sum  Inputs=++|
  Transpose1 : Math  Operator=transpose  SaturateOnIntegerOverflow=on
  alpha_dot : Outport
  wires:
  Direction Cosine Matrix Body to Wind/1 -> Transpose1/1
  Transpose1/1 -> Product1/1
  Product1/1 -> Selector2/1
  Selector2/1 -> Product2/1
  Selector3/1 -> Product2/2
  Product2/1 -> Sum/2
  alpha,beta/1 -> Direction Cosine Matrix Body to Wind/1
  q/1 -> Sum/1
  Sum/1 -> alpha_dot/1
  Ab/1 -> Product1/2
  Vw/1 -> Selector3/1

== system mainV02_36/LIBIS Plant/Propulsion/Variant_Motor_1/mappedMotor_1/ESC_1 ==
  V_battery : Inport  Unit=V
  Throttle : Inport  Port=2  Unit=1
  Product : Product
  Product1 : Product
  eta_ESC : Constant  Value=LD.Propulsion.ESC1.eta
  V_ESC : Outport  Unit=V
  wires:
  eta_ESC/1 -> Product/2
  V_battery/1 -> Product/1
  Product/1 -> Product1/1
  Product1/1 -> V_ESC/1
  Throttle/1 -> Product1/2

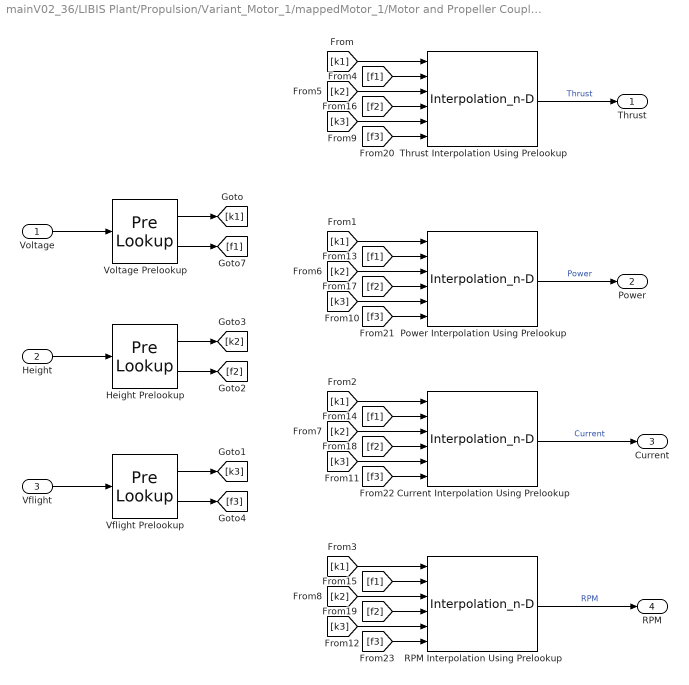
== system mainV02_36/LIBIS Plant/Propulsion/Variant_Motor_1/mappedMotor_1/Motor and Propeller Coupling_1 ==
  Voltage : Inport
  Height : Inport  Port=2
  Vflight : Inport  Port=3
  Current Interpolation Using Prelookup : Interpolation_n-D  NumberOfTableDimensions=3  Table=LD.Propulsion.motor1.Current  ExtrapMethod=Clip  DiagnosticForOutOfRangeInput=Warning  ValidIndexMayReachLast=on  InternalRulePriority=Speed
      settings: InputPortMap=u0,u1,u2,u3,u4,u5
  Height Prelookup : PreLookup  BreakpointsData=LD.Propulsion.motor1.Height  IndexSearchMethod=Evenly spaced points  BeginIndexSearchUsingPreviousIndexResult=on  UseLastBreakpoint=on
  Power Interpolation Using Prelookup : Interpolation_n-D  NumberOfTableDimensions=3  Table=LD.Propulsion.motor1.Power  ExtrapMethod=Clip  DiagnosticForOutOfRangeInput=Warning  ValidIndexMayReachLast=on  InternalRulePriority=Speed
      settings: InputPortMap=u0,u1,u2,u3,u4,u5
  RPM Interpolation Using Prelookup : Interpolation_n-D  NumberOfTableDimensions=3  Table=LD.Propulsion.motor1.RPM  ExtrapMethod=Clip  DiagnosticForOutOfRangeInput=Warning  ValidIndexMayReachLast=on  InternalRulePriority=Speed
      settings: InputPortMap=u0,u1,u2,u3,u4,u5
  Thrust Interpolation Using Prelookup : Interpolation_n-D  NumberOfTableDimensions=3  Table=LD.Propulsion.motor1.Thrust  ExtrapMethod=Clip  DiagnosticForOutOfRangeInput=Warning  ValidIndexMayReachLast=on  InternalRulePriority=Speed
      settings: InputPortMap=u0,u1,u2,u3,u4,u5
  Vflight Prelookup : PreLookup  BreakpointsData=LD.Propulsion.motor1.Vflight  IndexSearchMethod=Evenly spaced points  UseLastBreakpoint=on
  Voltage Prelookup : PreLookup  BreakpointsData=LD.Propulsion.motor1.Voltage  IndexSearchMethod=Evenly spaced points  UseLastBreakpoint=on
  Thrust : Outport
  Power : Outport  Port=2
  Current : Outport  Port=3
  RPM : Outport  Port=4
  wires:
  Height/1 -> Height Prelookup/1
  Vflight/1 -> Vflight Prelookup/1
  RPM Interpolation Using Prelookup/1 -> RPM/1  "RPM"
  Power Interpolation Using Prelookup/1 -> Power/1  "Power"
  Thrust Interpolation Using Prelookup/1 -> Thrust/1  "Thrust"
  Current Interpolation Using Prelookup/1 -> Current/1  "Current"
  Voltage/1 -> Voltage Prelookup/1
  Voltage Prelookup/1 -> [k1]
  Voltage Prelookup/2 -> [f1]
  Height Prelookup/1 -> [k2]
  Height Prelookup/2 -> [f2]
  Vflight Prelookup/2 -> [f3]
  Vflight Prelookup/1 -> [k3]
  [k1] -> Thrust Interpolation Using Prelookup/1
  [k1] -> Power Interpolation Using Prelookup/1
  [k1] -> Current Interpolation Using Prelookup/1
  [k1] -> RPM Interpolation Using Prelookup/1
  [f1] -> Thrust Interpolation Using Prelookup/2
  [k2] -> Thrust Interpolation Using Prelookup/3
  [k2] -> Power Interpolation Using Prelookup/3
  [k2] -> Current Interpolation Using Prelookup/3
  [k2] -> RPM Interpolation Using Prelookup/3
  [k3] -> Thrust Interpolation Using Prelookup/5
  [k3] -> Power Interpolation Using Prelookup/5
  [k3] -> Current Interpolation Using Prelookup/5
  [k3] -> RPM Interpolation Using Prelookup/5
  [f1] -> Power Interpolation Using Prelookup/2
  [f1] -> Current Interpolation Using Prelookup/2
  [f1] -> RPM Interpolation Using Prelookup/2
  [f2] -> RPM Interpolation Using Prelookup/4
  [f2] -> Current Interpolation Using Prelookup/4
  [f2] -> Power Interpolation Using Prelookup/4
  [f2] -> Thrust Interpolation Using Prelookup/4
  [f3] -> RPM Interpolation Using Prelookup/6
  [f3] -> Current Interpolation Using Prelookup/6
  [f3] -> Power Interpolation Using Prelookup/6
  [f3] -> Thrust Interpolation Using Prelookup/6

== system mainV02_36/LIBIS Plant/Propulsion/Variant_Motor_1/mappedMotor_1/Torque ==
  RPM : Inport
  Vflight : Inport  Port=2
  Constant : Constant  Value=1000
  Constant1 : Constant  Value=0
  RPM Prelookup : PreLookup  BreakpointsData=LD.Propulsion.propeller1.RPM(:,1)  IndexSearchMethod=Evenly spaced points  UseLastBreakpoint=on
  RPM1 : InportShadow
  Sum : Sum  Inputs=|-+
  Switch : Switch
  Torque Interpolation Using Prelookup : Interpolation_n-D  Table=LD.Propulsion.propeller1.Torque  ExtrapMethod=Clip  ValidIndexMayReachLast=on  InternalRulePriority=Speed
  Vflight Prelookup : PreLookup  BreakpointsData=LD.Propulsion.propeller1.V(1,:)  UseLastBreakpoint=on
  Torque : Outport
  wires:
  [k2] -> Torque Interpolation Using Prelookup/3
  RPM Prelookup/1 -> [k1]
  RPM Prelookup/2 -> [f1]
  [f1] -> Torque Interpolation Using Prelookup/2
  [k1] -> Torque Interpolation Using Prelookup/1
  [f2] -> Torque Interpolation Using Prelookup/4
  RPM/1 -> RPM Prelookup/1
  Vflight Prelookup/1 -> [k2]
  Vflight Prelookup/2 -> [f2]
  Vflight/1 -> Vflight Prelookup/1
  Torque Interpolation Using Prelookup/1 -> Switch/1  "Torque"
  Switch/1 -> Torque/1  "Torque"
  Sum/1 -> Switch/2
  Constant1/1 -> Switch/3
  Constant/1 -> Sum/1
  RPM1/1 -> Sum/2

== system mainV02_36/LIBIS Plant/Propulsion/Variant_Motor_1/noMappedMotor_1/ESC_1 ==
  V_battery : Inport  Unit=V
  Throttle : Inport  Port=2  Unit=1
  Product : Product
  Product1 : Product
  eta_ESC : Constant  Value=LD.Propulsion.ESC1.eta
  V_ESC : Outport  Unit=V
  wires:
  eta_ESC/1 -> Product/2
  V_battery/1 -> Product/1
  Product/1 -> Product1/1
  Product1/1 -> V_ESC/1
  Throttle/1 -> Product1/2

== system mainV02_36/LIBIS Plant/Propulsion/Variant_Motor_1/noMappedMotor_1/Motor_1 ==
  V_ESC : Inport
  Im : Inport  Port=2
  ActiveMotor1 : Subsystem  VariantControl=Variants.Motor2~=0
  Constant : Constant  Value=LD.Propulsion.motor1.I0
  Constant1 : Constant  Value=LD.Propulsion.motor1.Rm
  Peje Switch : Switch  Criteria=u2 > Threshold
  Product : Product
  RPM Switch : Switch  Criteria=u2 > Threshold
  Sum : Sum  Inputs=|+-
  V_ESC1 : InportShadow
  noActiveMotor1 : Subsystem  VariantControl=Variants.Motor2==0
  RPM : Outport
  Peje : Outport  Port=2
  wires:
  V_ESC/1 -> noActiveMotor1/1(V_ESC), ActiveMotor1/1(V_ESC)
  Im/1 -> noActiveMotor1/2(Im), ActiveMotor1/2(Im)
  Sum/1 -> Peje Switch/2, RPM Switch/2
  Peje Switch/1 -> Peje/1
  RPM Switch/1 -> RPM/1
  ActiveMotor1/1(RPM) -> RPM Switch/1
  noActiveMotor1/1(RPM) -> RPM Switch/3
  noActiveMotor1/2(Peje) -> Peje Switch/3
  ActiveMotor1/2(Peje) -> Peje Switch/1
  V_ESC1/1 -> Sum/1
  Product/1 -> Sum/2
  Constant/1 -> Product/1
  Constant1/1 -> Product/2

== system mainV02_36/LIBIS Plant/Propulsion/Variant_Motor_1/noMappedMotor_1/Propeller_1 ==
  RPM : Inport
  V_flight : Inport  Port=2
  airDensity : Inport  Port=3
  Constant : Constant  Value=5
  Constant1 : Constant  Value=3
  Constant2 : Constant  Value=4
  Constant3 : Constant  Value=2
  Cp Interpolation Using Prelookup : Interpolation_n-D  Table=LD.Propulsion.propeller1.Cp  ExtrapMethod=Clip  ValidIndexMayReachLast=on  InternalRulePriority=Speed
  Ct Interpolation Using Prelookup2 : Interpolation_n-D  Table=LD.Propulsion.propeller1.Ct  ExtrapMethod=Clip  ValidIndexMayReachLast=on  InternalRulePriority=Speed
  Diameter : Constant  Value=LD.Propulsion.propeller1.Diameter
  Gain : Gain  Gain=1/60
  Math Function{,1..3} (4 alike) : Math  Operator=pow  SaturateOnIntegerOverflow=on
  Prelookup4 : PreLookup  BreakpointsData=LD.Propulsion.propeller1.RPM  IndexSearchMethod=Evenly spaced points  UseLastBreakpoint=on
  Prelookup5 : PreLookup  BreakpointsData=LD.Propulsion.propeller1.V  UseLastBreakpoint=on
  Product : Product  Inputs=4
  Product1 : Product  Inputs=4
  RPM1 : InportShadow
  P_needed : Outport
  Thrust : Outport  Port=2
  wires:
  Diameter/1 -> Math Function2/1, Math Function/1  "D"
  Constant/1 -> Math Function/2  "5"
  Constant1/1 -> Math Function1/2  "3"
  Cp Interpolation Using Prelookup/1 -> Product/4  "Cp"
  Math Function1/1 -> Product/3  "n^3"
  Math Function/1 -> Product/2  "D^5"
  airDensity/1 -> Product/1, Product1/4  "airDensity"
  Product/1 -> P_needed/1  "Pneeded"
  Product1/1 -> Thrust/1  "Thrust"
  V_flight/1 -> Prelookup5/1  "V_flight"
  Constant2/1 -> Math Function2/2  "4"
  Math Function2/1 -> Product1/3  "D^4"
  Prelookup4/1 -> Cp Interpolation Using Prelookup/1, Ct Interpolation Using Prelookup2/1
  Prelookup4/2 -> Cp Interpolation Using Prelookup/2, Ct Interpolation Using Prelookup2/2
  Prelookup5/1 -> Cp Interpolation Using Prelookup/3, Ct Interpolation Using Prelookup2/3
  Prelookup5/2 -> Cp Interpolation Using Prelookup/4, Ct Interpolation Using Prelookup2/4
  Ct Interpolation Using Prelookup2/1 -> Product1/1  "Ct"
  Constant3/1 -> Math Function3/2  "2"
  Gain/1 -> Math Function1/1, Math Function3/1  "n_rev_s"
  Math Function3/1 -> Product1/2  "n^2"
  RPM1/1 -> Gain/1  "RPM"
  RPM/1 -> Prelookup4/1  "RPM"

== system mainV02_36/LIBIS Plant/Propulsion/Variant_Motor_1/noMappedMotor_1/Torque ==
  RPM : Inport
  Vflight : Inport  Port=2
  Constant : Constant  Value=1000
  Constant1 : Constant  Value=0
  RPM Prelookup : PreLookup  BreakpointsData=LD.Propulsion.propeller1.RPM(:,1)  IndexSearchMethod=Evenly spaced points  UseLastBreakpoint=on
  RPM1 : InportShadow
  Sum : Sum  Inputs=|-+
  Switch : Switch
  Torque Interpolation Using Prelookup : Interpolation_n-D  Table=LD.Propulsion.propeller1.Torque  ExtrapMethod=Clip  ValidIndexMayReachLast=on  InternalRulePriority=Speed
  Vflight Prelookup : PreLookup  BreakpointsData=LD.Propulsion.propeller1.V(1,:)  UseLastBreakpoint=on
  Torque : Outport
  wires:
  [k2] -> Torque Interpolation Using Prelookup/3
  RPM Prelookup/1 -> [k1]
  RPM Prelookup/2 -> [f1]
  [f1] -> Torque Interpolation Using Prelookup/2
  [k1] -> Torque Interpolation Using Prelookup/1
  [f2] -> Torque Interpolation Using Prelookup/4
  RPM/1 -> RPM Prelookup/1
  Vflight Prelookup/1 -> [k2]
  Vflight Prelookup/2 -> [f2]
  Vflight/1 -> Vflight Prelookup/1
  Torque Interpolation Using Prelookup/1 -> Switch/1  "Torque"
  Switch/1 -> Torque/1  "Torque"
  Sum/1 -> Switch/2
  Constant1/1 -> Switch/3
  Constant/1 -> Sum/1
  RPM1/1 -> Sum/2

== system mainV02_36/LIBIS Plant/Propulsion/Variant_Motor_2/mappedMotor_2/ESC_2 ==
  V_battery : Inport  Unit=V
  Throttle : Inport  Port=2  Unit=1
  Product : Product
  Product1 : Product
  eta_ESC : Constant  Value=LD.Propulsion.ESC2.eta
  V_ESC : Outport  Unit=V
  wires:
  eta_ESC/1 -> Product/2
  V_battery/1 -> Product/1
  Product/1 -> Product1/1
  Product1/1 -> V_ESC/1
  Throttle/1 -> Product1/2
